simulink model "relaying"  (Simulink 3.00)
settings: Solver=ode45  StartTime=0.0  StopTime=10.0  RelTol=1e-3
values from neighbouring files (symbols this model uses):
  den = [1]    [dab1.m]    (also in dab1o.m)
  dx = 0    [dab1.m]    (also in dab1o.m)
  num = [1]    [dab1.m]    (also in dab1o.m)
undefined symbols (not defined in the file or in its folder): aux, Time
libraries: ELEMENTS x5

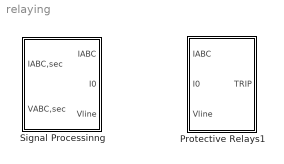
== system relaying ==
  Protective Relays1 : Subsystem
  Signal Processinng : Subsystem

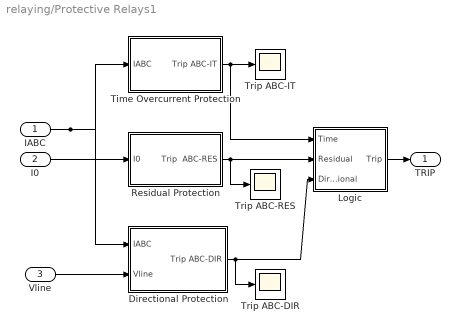
== system relaying/Protective Relays1 ==
  IABC : Inport  Port=1  PortWidth=-1  SampleTime=-1  DataType=auto
      settings: SignalType=auto
  I0 : Inport  Port=2  PortWidth=-1  SampleTime=-1  DataType=auto
      settings: SignalType=auto
  Vline : Inport  Port=3  PortWidth=-1  SampleTime=-1  DataType=auto
      settings: SignalType=auto
  Directional Protection : Subsystem  mask(Directional Elements){AA=-60, AB=120}
      mask prompts: AA "Angle alpha (deg)"; AB "Angle Beta (deg)"
  Logic : Subsystem
  Residual Protection : Subsystem
  Time Overcurrent Protection : Subsystem  mask(Overcurrent Protection){typed=Very Inverse, Pick=1.5, k=0.05}
      mask prompts: typed "Type of time dependency"; Pick "Pickup value:"; k "Time parameter (seconds):"
      mask init:
      | switch typed
      | case 1,
      |    string='Time defined';
      | case 2,
      |    string='Standard Inverse';
      | case 3,
      |    string='Very Inverse';
      | case 4,
      |    string='Extra Inverse';
      | case 5,
      |    string='RI Inverse';
      | case 6,
      |    string='Long Time Inverse';
      | end;
      | set_param('systemtotal/Protective Relays/Time Overcurrent Protection/UC1',...
      |    'Type1',string);
      | set_param('systemtotal/Protective Relays/Time Overcurrent Protection/UC2',...
      |    'Type1',string);
      | set_param('systemtotal/Protective Relays/Time Overcurrent Protection/UC3',...
      |    'Type1',string);
      mask StyleString: popup(Time defined|Standard Inverse|Very Inverse|Extra Inverse|RI Inverse|Long Time Inverse),edit,edit
  Trip ABC-DIR : Scope
      settings: TickLabels=on  TimeRange=auto  YMin=-1  YMax=1  SaveToWorkspace=off  SaveName=ScopeData  DataFormat=Matrix  LimitMaxRows=off
  Trip ABC-IT : Scope
      settings: TickLabels=on  TimeRange=auto  YMin=-1  YMax=1  SaveToWorkspace=off  SaveName=ScopeData  DataFormat=Matrix  LimitMaxRows=off
  Trip ABC-RES : Scope
      settings: TickLabels=on  TimeRange=auto  YMin=-1  YMax=1  SaveToWorkspace=off  SaveName=ScopeData  DataFormat=Matrix  LimitMaxRows=off
  TRIP : Outport  Port=1  InitialOutput=0
  wires:
  Vline/1 -> Directional Protection/2(Vline)
  I0/1 -> Residual Protection/1(I0)
  Logic/1(Trip) -> TRIP/1
  Directional Protection/1(Trip ABC-DIR) -> Logic/3(Directional), Trip ABC-DIR/1
  Time Overcurrent Protection/1(Trip ABC-IT) -> Logic/1(Time), Trip ABC-IT/1
  Residual Protection/1(Trip  ABC-RES) -> Logic/2(Residual), Trip ABC-RES/1
  IABC/1 -> Directional Protection/1(IABC), Time Overcurrent Protection/1(IABC)

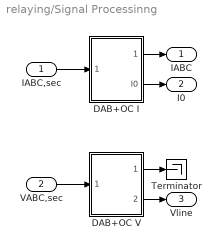
== system relaying/Signal Processinng ==
  IABC,sec : Inport  Port=1  PortWidth=-1  SampleTime=-1  DataType=auto
      settings: SignalType=auto
  VABC,sec : Inport  Port=2  PortWidth=-1  SampleTime=-1  DataType=auto
      settings: SignalType=auto
  DAB+OC I : Subsystem
  DAB+OC V : Subsystem
  Terminator : Terminator
  IABC : Outport  Port=1  InitialOutput=0
  I0 : Outport  Port=2  InitialOutput=0
  Vline : Outport  Port=3  InitialOutput=0
  wires:
  IABC,sec/1 -> DAB+OC I/1(IABC,sec)
  VABC,sec/1 -> DAB+OC V/1(VABC,sec)
  DAB+OC V/1(Vphase) -> Terminator/1
  DAB+OC I/1(IABC) -> IABC/1
  DAB+OC I/2(I0) -> I0/1
  DAB+OC V/2(Vline) -> Vline/1

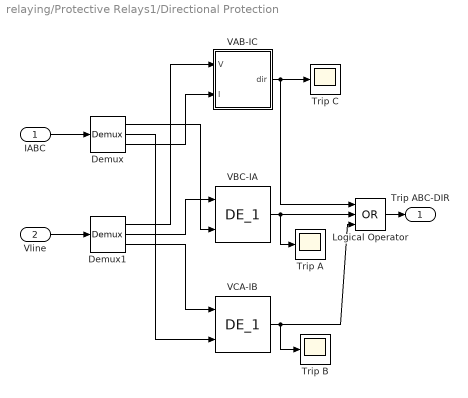
== system relaying/Protective Relays1/Directional Protection ==
  IABC : Inport  Port=1  PortWidth=-1  SampleTime=-1  DataType=auto
      settings: SignalType=auto
  Vline : Inport  Port=2  PortWidth=-1  SampleTime=-1  DataType=auto
      settings: SignalType=auto
  "  VAB-IC" : Subsystem  mask(Directional Element 1){alpha=AA, beta=AB, fs=40*60}
      mask prompts: alpha "Angle alpha [deg]"; beta "Angle Beta [deg]"; fs "Sampling frecuency (Hz):"
      mask help: This block has two phasor inputs: voltage and current. The operating characteristic is defined by two angles. The output is 1 when the current phasor falls into the operating characteristic.
      mask init:
      | DE_11;
      mask Help: web(['file:///' which('zc.html')]);
      mask Display: plot([0.2 0.8],[0.5 0.5],[0.5 0.6],[0.5 0.8],[0.5,xalpha],[0.5,yalpha],[0.5,xbeta],[0.5,ybeta]);
  "  VBC-IA" : ELEMENTS/  DE_1  alpha=AA  beta=AB  fs=40*60
  "  VCA-IB" : ELEMENTS/  DE_1  alpha=AA  beta=AB  fs=40*60
  Demux : Demux  Outputs=3
  Demux1 : Demux  Outputs=3
  Logical Operator : Logic  Operator=OR  Inputs=3
  Trip A : Scope
      settings: TickLabels=on  TimeRange=auto  YMin=-1  YMax=1  SaveToWorkspace=off  SaveName=ScopeData  DataFormat=Matrix  LimitMaxRows=off
  Trip B : Scope
      settings: TickLabels=on  TimeRange=auto  YMin=-1  YMax=1  SaveToWorkspace=off  SaveName=ScopeData  DataFormat=Matrix  LimitMaxRows=off
  Trip C : Scope
      settings: TickLabels=on  TimeRange=auto  YMin=-1  YMax=1  SaveToWorkspace=off  SaveName=ScopeData  DataFormat=Matrix  LimitMaxRows=off
  Trip ABC-DIR : Outport  Port=1  InitialOutput=0
  wires:
  "  VAB-IC"/1(dir) -> Logical Operator/1, Trip C/1
  "  VCA-IB"/1 -> Logical Operator/3, Trip B/1
  Demux1/3 -> "  VCA-IB"/1
  Demux/2 -> "  VCA-IB"/2
  Demux1/1 -> "  VAB-IC"/1(V)
  Demux/3 -> "  VAB-IC"/2(I)
  Demux1/2 -> "  VBC-IA"/1
  Demux/1 -> "  VBC-IA"/2
  Vline/1 -> Demux1/1
  IABC/1 -> Demux/1
  Logical Operator/1 -> Trip ABC-DIR/1
  "  VBC-IA"/1 -> Logical Operator/2, Trip A/1

== system relaying/Protective Relays1/Logic ==
  Time : Inport  Port=1  PortWidth=-1  SampleTime=-1  DataType=auto
      settings: SignalType=auto
  Residual : Inport  Port=2  PortWidth=-1  SampleTime=-1  DataType=auto
      settings: SignalType=auto
  Directional : Inport  Port=3  PortWidth=-1  SampleTime=-1  DataType=auto
      settings: SignalType=auto
  Logical Operator : Logic  Operator=OR  Inputs=3
  Trip : Outport  Port=1  InitialOutput=0
  wires:
  Directional/1 -> Logical Operator/3
  Logical Operator/1 -> Trip/1
  Time/1 -> Logical Operator/1
  Residual/1 -> Logical Operator/2

== system relaying/Protective Relays1/Residual Protection ==
  I0 : Inport  Port=1  PortWidth=-1  SampleTime=-1  DataType=auto
      settings: SignalType=auto
  Demux1 : Demux  Outputs=2
  UC1 : ELEMENTS/UC  type0=Signal-Time  sign=<  Ipickup=1.5  k1=1  type1=RI Inverse  type3=integration  k=0.05  fs=40*60
  Trip  ABC-RES : Outport  Port=1  InitialOutput=0
  wires:
  UC1/1 -> Trip  ABC-RES/1
  Demux1/2 -> UC1/2
  Demux1/1 -> UC1/1
  I0/1 -> Demux1/1

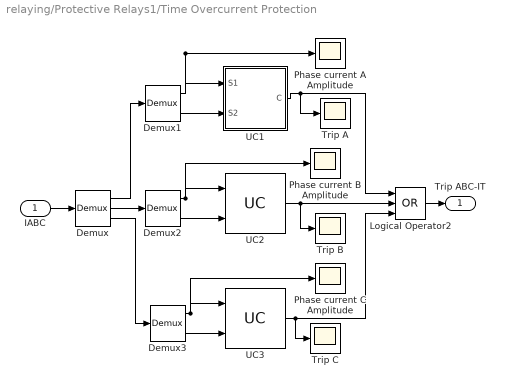
== system relaying/Protective Relays1/Time Overcurrent Protection ==
  IABC : Inport  Port=1  PortWidth=-1  SampleTime=-1  DataType=auto
      settings: SignalType=auto
  Demux : Demux  Outputs=3
  Demux1 : Demux  Outputs=2
  Demux2 : Demux  Outputs=2
  Demux3 : Demux  Outputs=2
  Logical Operator2 : Logic  Operator=OR  Inputs=3
  Phase current A Amplitude : Scope
      settings: TickLabels=on  TimeRange=auto  YMin=-1  YMax=1.25  SaveToWorkspace=off  SaveName=ScopeData  DataFormat=Matrix  LimitMaxRows=off
  Phase current B Amplitude : Scope
      settings: TickLabels=on  TimeRange=0.2  YMin=-1.25  YMax=1.25  SaveToWorkspace=off  SaveName=ScopeData  DataFormat=Matrix  LimitMaxRows=off
  Phase current C Amplitude : Scope
      settings: TickLabels=on  TimeRange=0.2  YMin=-20  YMax=30  SaveToWorkspace=off  SaveName=ScopeData  DataFormat=Matrix  LimitMaxRows=off
  Trip A : Scope
      settings: TickLabels=on  TimeRange=auto  YMin=0  YMax=1  SaveToWorkspace=off  SaveName=ScopeData  DataFormat=Matrix  LimitMaxRows=off
  Trip B : Scope
      settings: TickLabels=on  TimeRange=auto  YMin=0  YMax=1  SaveToWorkspace=off  SaveName=ScopeData  DataFormat=Matrix  LimitMaxRows=off
  Trip C : Scope
      settings: TickLabels=on  TimeRange=auto  YMin=0  YMax=1  SaveToWorkspace=off  SaveName=ScopeData  DataFormat=Matrix  LimitMaxRows=off
  UC1 : Subsystem  mask(Universal Comparator){type0=Signal-Time, sign=<, Ipickup=Pick, k1=1, type1=Very Inverse, type3=integration, k=k, fs=40*60}
      mask prompts: type0 "Type of comparison"; Ipickup "Pick-up value:"; k1 "Ratio of reset to pick-up:"; type1 "Type of Time dependency"; type3 "I-t emulation method"; k "Time parameter (seconds):"; fs "Sampling frequency (Hz):"
      mask help: This block is fed by two signals and does comparisons of three types: signal-to-signal, signal-to-threshold and signal-to-time. The options include the sign of the comparison, pick-up to re-set ratio, and the way of emulating the steady-state current characteristic.
      mask init:
      | uc0;
      mask Help: web(['file:///' which('uc.html')]);
      mask StyleString: popup(Signal-Threshold|Signal-Signal|Signal-Time),popup(>|<),edit,edit,popup(Time defined|Standard Inverse|Very Inverse|Extra Inverse|RI Inverse|Long Time Inverse),popup(Present value|integration),edit,edit
      mask Display:
      | disp(icon);
      | plot(current,time);
  UC2 : ELEMENTS/UC  type0=Signal-Time  sign=<  Ipickup=Pick  k1=1  type1=Very Inverse  type3=integration  k=k  fs=40*60
  UC3 : ELEMENTS/UC  type0=Signal-Time  sign=<  Ipickup=Pick  k1=1  type1=Very Inverse  type3=integration  k=k  fs=40*60
  Trip ABC-IT : Outport  Port=1  InitialOutput=0
  wires:
  UC1/1(C) -> Trip A/1, Logical Operator2/1
  IABC/1 -> Demux/1
  Demux/3 -> Demux3/1
  Demux/1 -> Demux1/1
  Demux/2 -> Demux2/1
  Logical Operator2/1 -> Trip ABC-IT/1
  Demux3/2 -> UC3/2
  Demux2/2 -> UC2/2
  Demux1/2 -> UC1/2(S2)
  UC3/1 -> Logical Operator2/3, Trip C/1
  UC2/1 -> Logical Operator2/2, Trip B/1
  Demux3/1 -> Phase current C Amplitude/1, UC3/1
  Demux2/1 -> Phase current B Amplitude/1, UC2/1
  Demux1/1 -> Phase current A Amplitude/1, UC1/1(S1)

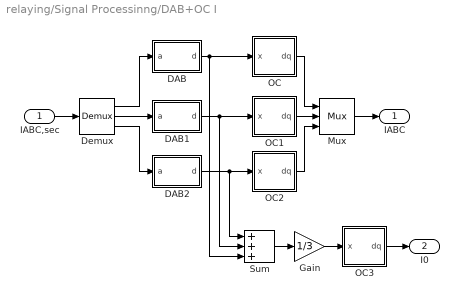
== system relaying/Signal Processinng/DAB+OC I ==
  IABC,sec : Inport  Port=1  PortWidth=-1  SampleTime=-1  DataType=auto
      settings: SignalType=auto
  DAB : Subsystem  mask(Data Adquisition Board){filter=off, approx=Bessel, order=2, numerator=[], denominator=[], freq=180, resdis=off, vertres=12, xmax=10, winsize=40, G=1.0, fs=60*40}
      mask prompts: filter "Disable Analog Filter"; approx "Filter approximation"; numerator "Free expression filter: numerator(descending order of s)"; denominator "Free expression filter: denominator:"; freq "Cut-off frequency"; resdis "Disable Vertical Resolution"; vertres "Vertical Resolution: No. of bits"; xmax "Vertical Resolution: signal range"; winsize "Window size"; G "Gain"; fs "Sampling frequency"
      mask help: Performs analog filtering, signal conditioning and sampling. A single signal is the input, a buffer with the signal samples is the output. The options include analog filter enable/disable switch, type, order and cut-off frequency of the analog filter, conditioning gain, sampling frequency, number of bits, the length of the buffer.
      mask init:
      | dab1
      mask Help: web(['file:///' which('dab.html')]);
      mask StyleString: checkbox,popup(Bessel|Tschebyscheff|Butterworth|free expression),popup(2|3|4),edit,edit,edit,checkbox,popup(8|12|16),edit,edit,edit,edit
      mask Display: disp('DAB')
  DAB1 : Subsystem  mask(Data Adquisition Board){filter=off, approx=Bessel, order=2, numerator=[], denominator=[], freq=180, resdis=off, vertres=12, xmax=10, winsize=40, G=1.0, fs=60*40}
      mask prompts: filter "Disable Analog Filter"; approx "Filter approximation"; numerator "Free expression filter: numerator(descending order of s)"; denominator "Free expression filter: denominator:"; freq "Cut-off frequency"; resdis "Disable Vertical Resolution"; vertres "Vertical Resolution: No. of bits"; xmax "Vertical Resolution: signal range"; winsize "Window size"; G "Gain"; fs "Sampling frequency"
      mask help: Performs analog filtering, signal conditioning and sampling. A single signal is the input, a buffer with the signal samples is the output. The options include analog filter enable/disable switch, type, order and cut-off frequency of the analog filter, conditioning gain, sampling frequency, number of bits, the length of the buffer.
      mask init:
      | dab1
      mask Help: web(['file:///' which('dab.html')]);
      mask StyleString: checkbox,popup(Bessel|Tschebyscheff|Butterworth|free expression),popup(2|3|4),edit,edit,edit,checkbox,popup(8|12|16),edit,edit,edit,edit
      mask Display: disp('DAB')
  DAB2 : Subsystem  mask(Data Adquisition Board){filter=off, approx=Bessel, order=2, numerator=[], denominator=[], freq=180, resdis=off, vertres=12, xmax=10, winsize=40, G=1.0, fs=60*40}
      mask prompts: filter "Disable Analog Filter"; approx "Filter approximation"; numerator "Free expression filter: numerator(descending order of s)"; denominator "Free expression filter: denominator:"; freq "Cut-off frequency"; resdis "Disable Vertical Resolution"; vertres "Vertical Resolution: No. of bits"; xmax "Vertical Resolution: signal range"; winsize "Window size"; G "Gain"; fs "Sampling frequency"
      mask help: Performs analog filtering, signal conditioning and sampling. A single signal is the input, a buffer with the signal samples is the output. The options include analog filter enable/disable switch, type, order and cut-off frequency of the analog filter, conditioning gain, sampling frequency, number of bits, the length of the buffer.
      mask init:
      | dab1
      mask Help: web(['file:///' which('dab.html')]);
      mask StyleString: checkbox,popup(Bessel|Tschebyscheff|Butterworth|free expression),popup(2|3|4),edit,edit,edit,checkbox,popup(8|12|16),edit,edit,edit,edit
      mask Display: disp('DAB')
  Demux : Demux  Outputs=3
  Gain : Gain  Gain=1/3  SaturateOnIntegerOverflow=on
  Mux : Mux  Inputs=3
      settings: DisplayOption=none
  OC : Subsystem  mask(Orthogonal Components){tfilt=Fourier, rfilt=[ ], ifilt=[ ], tlen=half, N1=40}
      mask prompts: tfilt "Type of filter:"; rfilt "Direct filter"; ifilt "Quadrature filter"; tlen "Type of data window"; N1 "Number of samples per cycle:"
      mask help: The block captures the data window of a sampled signal and computes the orthogonal components of the signal, i.e. amplitude and angle. The pre-defined filters include Fourier and Walsh functions. The free expression filters may also be used. Note: The type of data window affects only the Fourier filter.
      mask init:
      | oc2;
      mask Help:
      | This block take the date as its input window of the sampled signal, and convert it into a single orthogonal output. The output values are direct and quadrature orthogonal components of signal at the present sampling instant.
      | The options of the block include type and data window length of pre-defined filters and user-defined filters.
      mask StyleString: popup(Fourier|Walsh|User Defined),edit,edit,popup(half|full),edit
      mask Display: disp(DIFI);
  OC1 : Subsystem  mask(Orthogonal Components){tfilt=Fourier, rfilt=[ ], ifilt=[ ], tlen=half, N1=40}
      mask prompts: tfilt "Type of filter:"; rfilt "Direct filter"; ifilt "Quadrature filter"; tlen "Type of data window"; N1 "Number of samples per cycle:"
      mask help: The block captures the data window of a sampled signal and computes the orthogonal components of the signal, i.e. amplitude and angle. The pre-defined filters include Fourier and Walsh functions. The free expression filters may also be used. Note: The type of data window affects only the Fourier filter.
      mask init:
      | oc2;
      mask Help:
      | This block take the date as its input window of the sampled signal, and convert it into a single orthogonal output. The output values are direct and quadrature orthogonal components of signal at the present sampling instant.
      | The options of the block include type and data window length of pre-defined filters and user-defined filters.
      mask StyleString: popup(Fourier|Walsh|User Defined),edit,edit,popup(half|full),edit
      mask Display: disp(DIFI);
  OC2 : Subsystem  mask(Orthogonal Components){tfilt=Fourier, rfilt=[ ], ifilt=[ ], tlen=half, N1=40}
      mask prompts: tfilt "Type of filter:"; rfilt "Direct filter"; ifilt "Quadrature filter"; tlen "Type of data window"; N1 "Number of samples per cycle:"
      mask help: The block captures the data window of a sampled signal and computes the orthogonal components of the signal, i.e. amplitude and angle. The pre-defined filters include Fourier and Walsh functions. The free expression filters may also be used. Note: The type of data window affects only the Fourier filter.
      mask init:
      | oc2;
      mask Help:
      | This block take the date as its input window of the sampled signal, and convert it into a single orthogonal output. The output values are direct and quadrature orthogonal components of signal at the present sampling instant.
      | The options of the block include type and data window length of pre-defined filters and user-defined filters.
      mask StyleString: popup(Fourier|Walsh|User Defined),edit,edit,popup(half|full),edit
      mask Display: disp(DIFI);
  OC3 : Subsystem  mask(Orthogonal Components){tfilt=Fourier, rfilt=[ ], ifilt=[ ], tlen=half, N1=40}
      mask prompts: tfilt "Type of filter:"; rfilt "Direct filter"; ifilt "Quadrature filter"; tlen "Type of data window"; N1 "Number of samples per cycle:"
      mask help: The block captures the data window of a sampled signal and computes the orthogonal components of the signal, i.e. amplitude and angle. The pre-defined filters include Fourier and Walsh functions. The free expression filters may also be used. Note: The type of data window affects only the Fourier filter.
      mask init:
      | oc2;
      mask Help:
      | This block take the date as its input window of the sampled signal, and convert it into a single orthogonal output. The output values are direct and quadrature orthogonal components of signal at the present sampling instant.
      | The options of the block include type and data window length of pre-defined filters and user-defined filters.
      mask StyleString: popup(Fourier|Walsh|User Defined),edit,edit,popup(half|full),edit
      mask Display: disp(DIFI);
  Sum : Sum  Inputs=+++  SaturateOnIntegerOverflow=on
  IABC : Outport  Port=1  InitialOutput=0
  I0 : Outport  Port=2  InitialOutput=0
  wires:
  Demux/1 -> DAB/1(a)
  Demux/2 -> DAB1/1(a)
  Demux/3 -> DAB2/1(a)
  IABC,sec/1 -> Demux/1
  OC1/1(dq) -> Mux/2
  OC/1(dq) -> Mux/1
  OC2/1(dq) -> Mux/3
  Mux/1 -> IABC/1
  DAB2/1(d) -> OC2/1(x), Sum/1
  DAB1/1(d) -> OC1/1(x), Sum/2
  DAB/1(d) -> OC/1(x), Sum/3
  OC3/1(dq) -> I0/1
  Sum/1 -> Gain/1
  Gain/1 -> OC3/1(x)

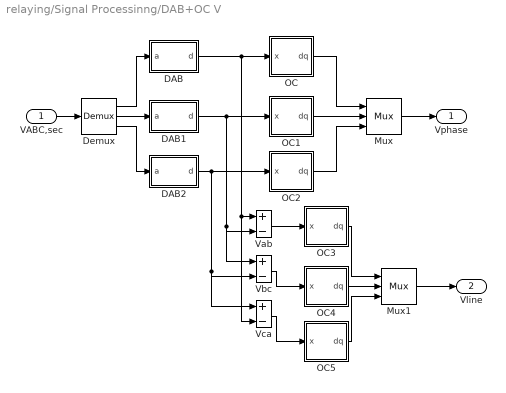
== system relaying/Signal Processinng/DAB+OC V ==
  VABC,sec : Inport  Port=1  PortWidth=-1  SampleTime=-1  DataType=auto
      settings: SignalType=auto
  DAB : Subsystem  mask(Data Adquisition Board){filter=off, approx=Bessel, order=2, numerator=[], denominator=[], freq=180, resdis=off, vertres=12, xmax=10, winsize=40, G=1.0, fs=60*40}
      mask prompts: filter "Disable Analog Filter"; approx "Filter approximation"; numerator "Free expression filter: numerator(descending order of s)"; denominator "Free expression filter: denominator:"; freq "Cut-off frequency"; resdis "Disable Vertical Resolution"; vertres "Vertical Resolution: No. of bits"; xmax "Vertical Resolution: signal range"; winsize "Window size"; G "Gain"; fs "Sampling frequency"
      mask help: Performs analog filtering, signal conditioning and sampling. A single signal is the input, a buffer with the signal samples is the output. The options include analog filter enable/disable switch, type, order and cut-off frequency of the analog filter, conditioning gain, sampling frequency, number of bits, the length of the buffer.
      mask init:
      | dab1
      mask Help: web(['file:///' which('dab.html')]);
      mask StyleString: checkbox,popup(Bessel|Tschebyscheff|Butterworth|free expression),popup(2|3|4),edit,edit,edit,checkbox,popup(8|12|16),edit,edit,edit,edit
      mask Display: disp('DAB')
  DAB1 : Subsystem  mask(Data Adquisition Board){filter=off, approx=Bessel, order=2, numerator=[], denominator=[], freq=180, resdis=off, vertres=12, xmax=10, winsize=40, G=1.0, fs=60*40}
      mask prompts: filter "Disable Analog Filter"; approx "Filter approximation"; numerator "Free expression filter: numerator(descending order of s)"; denominator "Free expression filter: denominator:"; freq "Cut-off frequency"; resdis "Disable Vertical Resolution"; vertres "Vertical Resolution: No. of bits"; xmax "Vertical Resolution: signal range"; winsize "Window size"; G "Gain"; fs "Sampling frequency"
      mask help: Performs analog filtering, signal conditioning and sampling. A single signal is the input, a buffer with the signal samples is the output. The options include analog filter enable/disable switch, type, order and cut-off frequency of the analog filter, conditioning gain, sampling frequency, number of bits, the length of the buffer.
      mask init:
      | dab1
      mask Help: web(['file:///' which('dab.html')]);
      mask StyleString: checkbox,popup(Bessel|Tschebyscheff|Butterworth|free expression),popup(2|3|4),edit,edit,edit,checkbox,popup(8|12|16),edit,edit,edit,edit
      mask Display: disp('DAB')
  DAB2 : Subsystem  mask(Data Adquisition Board){filter=off, approx=Bessel, order=2, numerator=[], denominator=[], freq=180, resdis=off, vertres=12, xmax=10, winsize=40, G=1.0, fs=60*40}
      mask prompts: filter "Disable Analog Filter"; approx "Filter approximation"; numerator "Free expression filter: numerator(descending order of s)"; denominator "Free expression filter: denominator:"; freq "Cut-off frequency"; resdis "Disable Vertical Resolution"; vertres "Vertical Resolution: No. of bits"; xmax "Vertical Resolution: signal range"; winsize "Window size"; G "Gain"; fs "Sampling frequency"
      mask help: Performs analog filtering, signal conditioning and sampling. A single signal is the input, a buffer with the signal samples is the output. The options include analog filter enable/disable switch, type, order and cut-off frequency of the analog filter, conditioning gain, sampling frequency, number of bits, the length of the buffer.
      mask init:
      | dab1
      mask Help: web(['file:///' which('dab.html')]);
      mask StyleString: checkbox,popup(Bessel|Tschebyscheff|Butterworth|free expression),popup(2|3|4),edit,edit,edit,checkbox,popup(8|12|16),edit,edit,edit,edit
      mask Display: disp('DAB')
  Demux : Demux  Outputs=3
  Mux : Mux  Inputs=3
      settings: DisplayOption=none
  Mux1 : Mux  Inputs=3
      settings: DisplayOption=none
  OC : Subsystem  mask(Orthogonal Components){tfilt=Fourier, rfilt=[ ], ifilt=[ ], tlen=half, N1=40}
      mask prompts: tfilt "Type of filter:"; rfilt "Direct filter"; ifilt "Quadrature filter"; tlen "Type of data window"; N1 "Number of samples per cycle:"
      mask help: The block captures the data window of a sampled signal and computes the orthogonal components of the signal, i.e. amplitude and angle. The pre-defined filters include Fourier and Walsh functions. The free expression filters may also be used. Note: The type of data window affects only the Fourier filter.
      mask init:
      | oc2;
      mask Help:
      | This block take the date as its input window of the sampled signal, and convert it into a single orthogonal output. The output values are direct and quadrature orthogonal components of signal at the present sampling instant.
      | The options of the block include type and data window length of pre-defined filters and user-defined filters.
      mask StyleString: popup(Fourier|Walsh|User Defined),edit,edit,popup(half|full),edit
      mask Display: disp(DIFI);
  OC1 : Subsystem  mask(Orthogonal Components){tfilt=Fourier, rfilt=[ ], ifilt=[ ], tlen=half, N1=40}
      mask prompts: tfilt "Type of filter:"; rfilt "Direct filter"; ifilt "Quadrature filter"; tlen "Type of data window"; N1 "Number of samples per cycle:"
      mask help: The block captures the data window of a sampled signal and computes the orthogonal components of the signal, i.e. amplitude and angle. The pre-defined filters include Fourier and Walsh functions. The free expression filters may also be used. Note: The type of data window affects only the Fourier filter.
      mask init:
      | oc2;
      mask Help:
      | This block take the date as its input window of the sampled signal, and convert it into a single orthogonal output. The output values are direct and quadrature orthogonal components of signal at the present sampling instant.
      | The options of the block include type and data window length of pre-defined filters and user-defined filters.
      mask StyleString: popup(Fourier|Walsh|User Defined),edit,edit,popup(half|full),edit
      mask Display: disp(DIFI);
  OC2 : Subsystem  mask(Orthogonal Components){tfilt=Fourier, rfilt=[ ], ifilt=[ ], tlen=half, N1=40}
      mask prompts: tfilt "Type of filter:"; rfilt "Direct filter"; ifilt "Quadrature filter"; tlen "Type of data window"; N1 "Number of samples per cycle:"
      mask help: The block captures the data window of a sampled signal and computes the orthogonal components of the signal, i.e. amplitude and angle. The pre-defined filters include Fourier and Walsh functions. The free expression filters may also be used. Note: The type of data window affects only the Fourier filter.
      mask init:
      | oc2;
      mask Help:
      | This block take the date as its input window of the sampled signal, and convert it into a single orthogonal output. The output values are direct and quadrature orthogonal components of signal at the present sampling instant.
      | The options of the block include type and data window length of pre-defined filters and user-defined filters.
      mask StyleString: popup(Fourier|Walsh|User Defined),edit,edit,popup(half|full),edit
      mask Display: disp(DIFI);
  OC3 : Subsystem  mask(Orthogonal Components){tfilt=Fourier, rfilt=[ ], ifilt=[ ], tlen=half, N1=40}
      mask prompts: tfilt "Type of filter:"; rfilt "Direct filter"; ifilt "Quadrature filter"; tlen "Type of data window"; N1 "Number of samples per cycle:"
      mask help: The block captures the data window of a sampled signal and computes the orthogonal components of the signal, i.e. amplitude and angle. The pre-defined filters include Fourier and Walsh functions. The free expression filters may also be used. Note: The type of data window affects only the Fourier filter.
      mask init:
      | oc2;
      mask Help:
      | This block take the date as its input window of the sampled signal, and convert it into a single orthogonal output. The output values are direct and quadrature orthogonal components of signal at the present sampling instant.
      | The options of the block include type and data window length of pre-defined filters and user-defined filters.
      mask StyleString: popup(Fourier|Walsh|User Defined),edit,edit,popup(half|full),edit
      mask Display: disp(DIFI);
  OC4 : Subsystem  mask(Orthogonal Components){tfilt=Fourier, rfilt=[ ], ifilt=[ ], tlen=half, N1=40}
      mask prompts: tfilt "Type of filter:"; rfilt "Direct filter"; ifilt "Quadrature filter"; tlen "Type of data window"; N1 "Number of samples per cycle:"
      mask help: The block captures the data window of a sampled signal and computes the orthogonal components of the signal, i.e. amplitude and angle. The pre-defined filters include Fourier and Walsh functions. The free expression filters may also be used. Note: The type of data window affects only the Fourier filter.
      mask init:
      | oc2;
      mask Help:
      | This block take the date as its input window of the sampled signal, and convert it into a single orthogonal output. The output values are direct and quadrature orthogonal components of signal at the present sampling instant.
      | The options of the block include type and data window length of pre-defined filters and user-defined filters.
      mask StyleString: popup(Fourier|Walsh|User Defined),edit,edit,popup(half|full),edit
      mask Display: disp(DIFI);
  OC5 : Subsystem  mask(Orthogonal Components){tfilt=Fourier, rfilt=[ ], ifilt=[ ], tlen=half, N1=40}
      mask prompts: tfilt "Type of filter:"; rfilt "Direct filter"; ifilt "Quadrature filter"; tlen "Type of data window"; N1 "Number of samples per cycle:"
      mask help: The block captures the data window of a sampled signal and computes the orthogonal components of the signal, i.e. amplitude and angle. The pre-defined filters include Fourier and Walsh functions. The free expression filters may also be used. Note: The type of data window affects only the Fourier filter.
      mask init:
      | oc2;
      mask Help:
      | This block take the date as its input window of the sampled signal, and convert it into a single orthogonal output. The output values are direct and quadrature orthogonal components of signal at the present sampling instant.
      | The options of the block include type and data window length of pre-defined filters and user-defined filters.
      mask StyleString: popup(Fourier|Walsh|User Defined),edit,edit,popup(half|full),edit
      mask Display: disp(DIFI);
  Vab : Sum  Inputs=+-  SaturateOnIntegerOverflow=on
  Vbc : Sum  Inputs=+-  SaturateOnIntegerOverflow=on
  Vca : Sum  Inputs=+-  SaturateOnIntegerOverflow=on
  Vphase : Outport  Port=1  InitialOutput=0
  Vline : Outport  Port=2
  wires:
  Demux/1 -> DAB/1(a)
  Demux/2 -> DAB1/1(a)
  Demux/3 -> DAB2/1(a)
  VABC,sec/1 -> Demux/1
  DAB/1(d) -> OC/1(x), Vab/1, Vca/2
  DAB1/1(d) -> OC1/1(x), Vab/2, Vbc/1
  DAB2/1(d) -> OC2/1(x), Vbc/2, Vca/1
  Vab/1 -> OC3/1(x)
  Vbc/1 -> OC4/1(x)
  Vca/1 -> OC5/1(x)
  OC1/1(dq) -> Mux/2
  OC/1(dq) -> Mux/1
  OC2/1(dq) -> Mux/3
  Mux/1 -> Vphase/1
  Mux1/1 -> Vline/1
  OC4/1(dq) -> Mux1/2
  OC3/1(dq) -> Mux1/1
  OC5/1(dq) -> Mux1/3

== system relaying/Protective Relays1/Directional Protection/  VAB-IC ==
  V : Inport  Port=1  PortWidth=-1  SampleTime=-1  DataType=auto
      settings: SignalType=auto
  I : Inport  Port=2  PortWidth=-1  SampleTime=-1  DataType=auto
      settings: SignalType=auto
  Mux : Mux  Inputs=2
      settings: DisplayOption=none
  S-Function : S-Function  FunctionName=DE_12  Parameters=alpha,beta,fs  PortCounts=[]  SFunctionModules=''
  dir : Outport  Port=1  InitialOutput=0
  wires:
  S-Function/1 -> dir/1
  Mux/1 -> S-Function/1
  V/1 -> Mux/1
  I/1 -> Mux/2

== system relaying/Protective Relays1/Time Overcurrent Protection/UC1 ==
  S1 : Inport  Port=1  PortWidth=-1  SampleTime=-1  DataType=auto
      settings: SignalType=auto
  S2 : Inport  Port=2  PortWidth=-1  SampleTime=-1  DataType=auto
      settings: SignalType=auto
  Mux : Mux  Inputs=2
      settings: DisplayOption=none
  S-Function : S-Function  FunctionName=uc1  Parameters=k,k1,aux,Ipickup,fs  PortCounts=[]  SFunctionModules=''
  C : Outport  Port=1  InitialOutput=0
  wires:
  S2/1 -> Mux/2
  S1/1 -> Mux/1
  Mux/1 -> S-Function/1
  S-Function/1 -> C/1

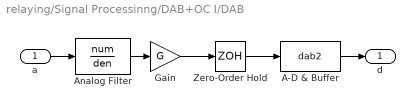
== system relaying/Signal Processinng/DAB+OC I/DAB ==
  a : Inport  Port=1  PortWidth=-1  SampleTime=-1  DataType=auto
      settings: SignalType=auto
  A-D & Buffer : S-Function  FunctionName=dab2  Parameters=winsize,fs,dx,resdis  PortCounts=[]  SFunctionModules=''
  Analog Filter : TransferFcn  Numerator=num  Denominator=den
  Gain : Gain  Gain=G  SaturateOnIntegerOverflow=on
  Zero-Order Hold : ZeroOrderHold  SampleTime=1/fs
  d : Outport  Port=1  InitialOutput=[zeros(winsize,1)]
  wires:
  A-D & Buffer/1 -> d/1
  a/1 -> Analog Filter/1
  Zero-Order Hold/1 -> A-D & Buffer/1
  Gain/1 -> Zero-Order Hold/1
  Analog Filter/1 -> Gain/1

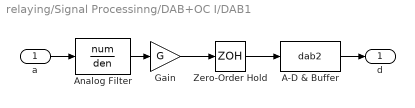
== system relaying/Signal Processinng/DAB+OC I/DAB1 ==
  a : Inport  Port=1  PortWidth=-1  SampleTime=-1  DataType=auto
      settings: SignalType=auto
  A-D & Buffer : S-Function  FunctionName=dab2  Parameters=winsize,fs,dx,resdis  PortCounts=[]  SFunctionModules=''
  Analog Filter : TransferFcn  Numerator=num  Denominator=den
  Gain : Gain  Gain=G  SaturateOnIntegerOverflow=on
  Zero-Order Hold : ZeroOrderHold  SampleTime=1/fs
  d : Outport  Port=1  InitialOutput=[zeros(winsize,1)]
  wires:
  A-D & Buffer/1 -> d/1
  a/1 -> Analog Filter/1
  Zero-Order Hold/1 -> A-D & Buffer/1
  Gain/1 -> Zero-Order Hold/1
  Analog Filter/1 -> Gain/1

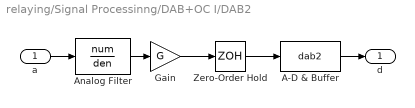
== system relaying/Signal Processinng/DAB+OC I/DAB2 ==
  a : Inport  Port=1  PortWidth=-1  SampleTime=-1  DataType=auto
      settings: SignalType=auto
  A-D & Buffer : S-Function  FunctionName=dab2  Parameters=winsize,fs,dx,resdis  PortCounts=[]  SFunctionModules=''
  Analog Filter : TransferFcn  Numerator=num  Denominator=den
  Gain : Gain  Gain=G  SaturateOnIntegerOverflow=on
  Zero-Order Hold : ZeroOrderHold  SampleTime=1/fs
  d : Outport  Port=1  InitialOutput=[zeros(winsize,1)]
  wires:
  A-D & Buffer/1 -> d/1
  a/1 -> Analog Filter/1
  Zero-Order Hold/1 -> A-D & Buffer/1
  Gain/1 -> Zero-Order Hold/1
  Analog Filter/1 -> Gain/1

== system relaying/Signal Processinng/DAB+OC I/OC ==
  note: v(t) is a vector
      | with width N1
  note: v_ort is
      | a complex number
  x : Inport  Port=1  PortWidth=-1  SampleTime=-1  DataType=auto
      settings: SignalType=auto
  OC filter : S-Function  FunctionName=oc1  Parameters=tfilt, rfilt, ifilt, tlen, N1  PortCounts=[]  SFunctionModules=''
  dq : Outport  Port=1  InitialOutput=0
  wires:
  x/1 -> OC filter/1
  OC filter/1 -> dq/1

== system relaying/Signal Processinng/DAB+OC I/OC1 ==
  note: v(t) is a vector
      | with width N1
  note: v_ort is
      | a complex number
  x : Inport  Port=1  PortWidth=-1  SampleTime=-1  DataType=auto
      settings: SignalType=auto
  OC filter : S-Function  FunctionName=oc1  Parameters=tfilt, rfilt, ifilt, tlen, N1  PortCounts=[]  SFunctionModules=''
  dq : Outport  Port=1  InitialOutput=0
  wires:
  x/1 -> OC filter/1
  OC filter/1 -> dq/1

== system relaying/Signal Processinng/DAB+OC I/OC2 ==
  note: v(t) is a vector
      | with width N1
  note: v_ort is
      | a complex number
  x : Inport  Port=1  PortWidth=-1  SampleTime=-1  DataType=auto
      settings: SignalType=auto
  OC filter : S-Function  FunctionName=oc1  Parameters=tfilt, rfilt, ifilt, tlen, N1  PortCounts=[]  SFunctionModules=''
  dq : Outport  Port=1  InitialOutput=0
  wires:
  x/1 -> OC filter/1
  OC filter/1 -> dq/1

== system relaying/Signal Processinng/DAB+OC I/OC3 ==
  note: v(t) is a vector
      | with width N1
  note: v_ort is
      | a complex number
  x : Inport  Port=1  PortWidth=-1  SampleTime=-1  DataType=auto
      settings: SignalType=auto
  OC filter : S-Function  FunctionName=oc1  Parameters=tfilt, rfilt, ifilt, tlen, N1  PortCounts=[]  SFunctionModules=''
  dq : Outport  Port=1  InitialOutput=0
  wires:
  x/1 -> OC filter/1
  OC filter/1 -> dq/1

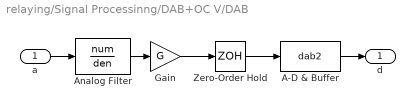
== system relaying/Signal Processinng/DAB+OC V/DAB ==
  a : Inport  Port=1  PortWidth=-1  SampleTime=-1  DataType=auto
      settings: SignalType=auto
  A-D & Buffer : S-Function  FunctionName=dab2  Parameters=winsize,fs,dx,resdis  PortCounts=[]  SFunctionModules=''
  Analog Filter : TransferFcn  Numerator=num  Denominator=den
  Gain : Gain  Gain=G  SaturateOnIntegerOverflow=on
  Zero-Order Hold : ZeroOrderHold  SampleTime=1/fs
  d : Outport  Port=1  InitialOutput=[zeros(winsize,1)]
  wires:
  A-D & Buffer/1 -> d/1
  a/1 -> Analog Filter/1
  Zero-Order Hold/1 -> A-D & Buffer/1
  Gain/1 -> Zero-Order Hold/1
  Analog Filter/1 -> Gain/1

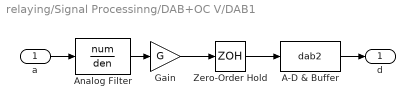
== system relaying/Signal Processinng/DAB+OC V/DAB1 ==
  a : Inport  Port=1  PortWidth=-1  SampleTime=-1  DataType=auto
      settings: SignalType=auto
  A-D & Buffer : S-Function  FunctionName=dab2  Parameters=winsize,fs,dx,resdis  PortCounts=[]  SFunctionModules=''
  Analog Filter : TransferFcn  Numerator=num  Denominator=den
  Gain : Gain  Gain=G  SaturateOnIntegerOverflow=on
  Zero-Order Hold : ZeroOrderHold  SampleTime=1/fs
  d : Outport  Port=1  InitialOutput=[zeros(winsize,1)]
  wires:
  A-D & Buffer/1 -> d/1
  a/1 -> Analog Filter/1
  Zero-Order Hold/1 -> A-D & Buffer/1
  Gain/1 -> Zero-Order Hold/1
  Analog Filter/1 -> Gain/1

== system relaying/Signal Processinng/DAB+OC V/DAB2 ==
  a : Inport  Port=1  PortWidth=-1  SampleTime=-1  DataType=auto
      settings: SignalType=auto
  A-D & Buffer : S-Function  FunctionName=dab2  Parameters=winsize,fs,dx,resdis  PortCounts=[]  SFunctionModules=''
  Analog Filter : TransferFcn  Numerator=num  Denominator=den
  Gain : Gain  Gain=G  SaturateOnIntegerOverflow=on
  Zero-Order Hold : ZeroOrderHold  SampleTime=1/fs
  d : Outport  Port=1  InitialOutput=[zeros(winsize,1)]
  wires:
  A-D & Buffer/1 -> d/1
  a/1 -> Analog Filter/1
  Zero-Order Hold/1 -> A-D & Buffer/1
  Gain/1 -> Zero-Order Hold/1
  Analog Filter/1 -> Gain/1

== system relaying/Signal Processinng/DAB+OC V/OC ==
  note: v(t) is a vector
      | with width N1
  note: v_ort is
      | a complex number
  x : Inport  Port=1  PortWidth=-1  SampleTime=-1  DataType=auto
      settings: SignalType=auto
  OC filter : S-Function  FunctionName=oc1  Parameters=tfilt, rfilt, ifilt, tlen, N1  PortCounts=[]  SFunctionModules=''
  dq : Outport  Port=1  InitialOutput=0
  wires:
  x/1 -> OC filter/1
  OC filter/1 -> dq/1

== system relaying/Signal Processinng/DAB+OC V/OC1 ==
  note: v(t) is a vector
      | with width N1
  note: v_ort is
      | a complex number
  x : Inport  Port=1  PortWidth=-1  SampleTime=-1  DataType=auto
      settings: SignalType=auto
  OC filter : S-Function  FunctionName=oc1  Parameters=tfilt, rfilt, ifilt, tlen, N1  PortCounts=[]  SFunctionModules=''
  dq : Outport  Port=1  InitialOutput=0
  wires:
  x/1 -> OC filter/1
  OC filter/1 -> dq/1

== system relaying/Signal Processinng/DAB+OC V/OC2 ==
  note: v(t) is a vector
      | with width N1
  note: v_ort is
      | a complex number
  x : Inport  Port=1  PortWidth=-1  SampleTime=-1  DataType=auto
      settings: SignalType=auto
  OC filter : S-Function  FunctionName=oc1  Parameters=tfilt, rfilt, ifilt, tlen, N1  PortCounts=[]  SFunctionModules=''
  dq : Outport  Port=1  InitialOutput=0
  wires:
  x/1 -> OC filter/1
  OC filter/1 -> dq/1

== system relaying/Signal Processinng/DAB+OC V/OC3 ==
  note: v(t) is a vector
      | with width N1
  note: v_ort is
      | a complex number
  x : Inport  Port=1  PortWidth=-1  SampleTime=-1  DataType=auto
      settings: SignalType=auto
  OC filter : S-Function  FunctionName=oc1  Parameters=tfilt, rfilt, ifilt, tlen, N1  PortCounts=[]  SFunctionModules=''
  dq : Outport  Port=1  InitialOutput=0
  wires:
  x/1 -> OC filter/1
  OC filter/1 -> dq/1

== system relaying/Signal Processinng/DAB+OC V/OC4 ==
  note: v(t) is a vector
      | with width N1
  note: v_ort is
      | a complex number
  x : Inport  Port=1  PortWidth=-1  SampleTime=-1  DataType=auto
      settings: SignalType=auto
  OC filter : S-Function  FunctionName=oc1  Parameters=tfilt, rfilt, ifilt, tlen, N1  PortCounts=[]  SFunctionModules=''
  dq : Outport  Port=1  InitialOutput=0
  wires:
  x/1 -> OC filter/1
  OC filter/1 -> dq/1

== system relaying/Signal Processinng/DAB+OC V/OC5 ==
  note: v(t) is a vector
      | with width N1
  note: v_ort is
      | a complex number
  x : Inport  Port=1  PortWidth=-1  SampleTime=-1  DataType=auto
      settings: SignalType=auto
  OC filter : S-Function  FunctionName=oc1  Parameters=tfilt, rfilt, ifilt, tlen, N1  PortCounts=[]  SFunctionModules=''
  dq : Outport  Port=1  InitialOutput=0
  wires:
  x/1 -> OC filter/1
  OC filter/1 -> dq/1
